simulink model "example_simulink_Manipulator"  (Simulink 7.0)
settings: Solver=FixedStepDiscrete  StartTime=0.0  StopTime=inf  FixedStep=20  RelTol=1e-3
libraries: lib_robotinohardware x3, simulink x1
settings Model: Creator=indorewala  LastModifiedBy=indorewala

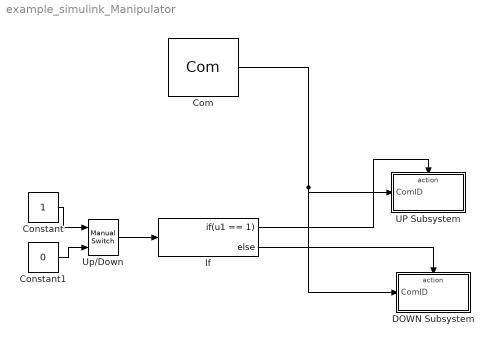
== system example_simulink_Manipulator ==
  Com : lib_robotinohardware/Com  ip='127.0.0.1'
  Constant : Constant  OutDataType=sfix(16)  OutScaling=2^0
  Constant1 : Constant  Value=0  OutDataType=sfix(16)  OutScaling=2^0
  DOWN Subsystem : Subsystem  TreatAsAtomicUnit=on
  If : If  IfExpression=u1 == 1
  UP Subsystem : Subsystem  TreatAsAtomicUnit=on
  Up/Down : simulink/Signal Routing/Manual Switch  SystemSampleTime=-1  sw=1  action=0  varsize=off
  wires:
  If/2 -> DOWN Subsystem/Action
  Com/1 -> UP Subsystem/1(ComID), DOWN Subsystem/1(ComID)
  Up/Down/1 -> If/1
  If/1 -> UP Subsystem/Action
  Constant/1 -> Up/Down/1
  Constant1/1 -> Up/Down/2

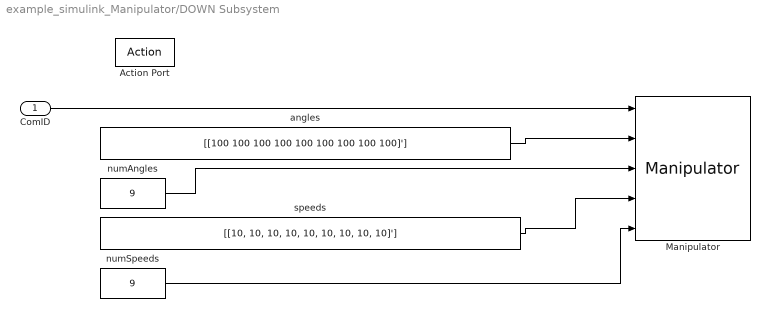
== system example_simulink_Manipulator/DOWN Subsystem ==
  ComID : Inport  OutDataType=sfix(16)  OutScaling=2^0
  Action Port : ActionPort  ActionType=else
  Manipulator : lib_robotinohardware/Manipulator
  angles : Constant  Value=[[100 100 100 100 100 100 100 100 100]']  VectorParams1D=off  OutDataTypeMode=single  OutDataType=sfix(16)  OutScaling=2^0
  numAngles : Constant  Value=9  OutDataTypeMode=uint32  OutDataType=sfix(16)  OutScaling=2^0
  numSpeeds : Constant  Value=9  OutDataTypeMode=uint32  OutDataType=sfix(16)  OutScaling=2^0
  speeds : Constant  Value=[[10, 10, 10, 10, 10, 10, 10, 10, 10]']  VectorParams1D=off  OutDataTypeMode=single  OutDataType=sfix(16)  OutScaling=2^0
  wires:
  angles/1 -> Manipulator/2
  numAngles/1 -> Manipulator/3
  speeds/1 -> Manipulator/4
  numSpeeds/1 -> Manipulator/5
  ComID/1 -> Manipulator/1

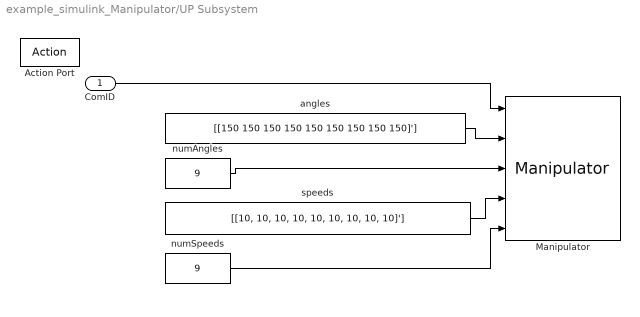
== system example_simulink_Manipulator/UP Subsystem ==
  ComID : Inport  OutDataType=sfix(16)  OutScaling=2^0
  Action Port : ActionPort  ActionType=then
  Manipulator : lib_robotinohardware/Manipulator
  angles : Constant  Value=[[150 150 150 150 150 150 150 150 150]']  VectorParams1D=off  OutDataTypeMode=single  OutDataType=sfix(16)  OutScaling=2^0
  numAngles : Constant  Value=9  OutDataTypeMode=uint32  OutDataType=sfix(16)  OutScaling=2^0
  numSpeeds : Constant  Value=9  OutDataTypeMode=uint32  OutDataType=sfix(16)  OutScaling=2^0
  speeds : Constant  Value=[[10, 10, 10, 10, 10, 10, 10, 10, 10]']  VectorParams1D=off  OutDataTypeMode=single  OutDataType=sfix(16)  OutScaling=2^0
  wires:
  angles/1 -> Manipulator/2
  numAngles/1 -> Manipulator/3
  speeds/1 -> Manipulator/4
  numSpeeds/1 -> Manipulator/5
  ComID/1 -> Manipulator/1
